simulink model "controllore2_nonlineare_con_gravita"  (R2022b)
settings: Solver=VariableStepAuto  StartTime=0.0  StopTime=10.0  RelTol=1e-3
settings Model: Creator=Antonio Montalto  LastModifiedBy=natal

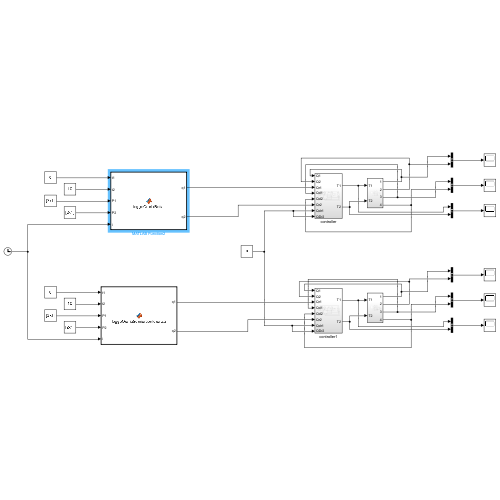
[thumbnail: Simulink's stored preview of the top-level diagram]
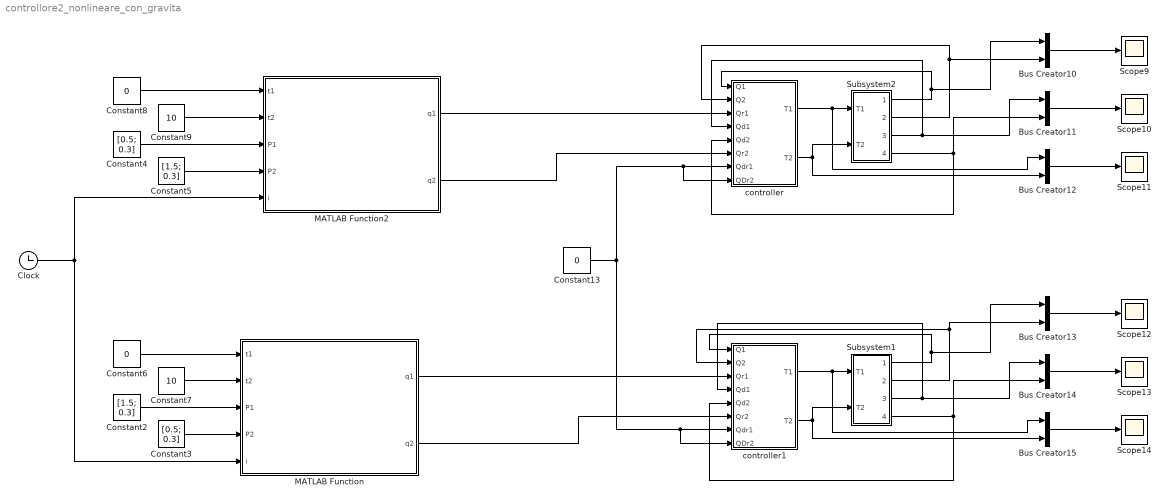
== system controllore2_nonlineare_con_gravita ==
  Bus Creator{10..15} (6 alike) : BusCreator  Inputs=2
  Clock : Clock
      settings: Decimation=1000
  Constant13 : Constant  Value=0
  Constant2 : Constant  Value=[1.5; 0.3]
  Constant3 : Constant  Value=[0.5; 0.3]
  Constant4 : Constant  Value=[0.5; 0.3]
  Constant5 : Constant  Value=[1.5; 0.3]
  Constant6 : Constant  Value=0
  Constant7 : Constant  Value=10
  Constant8 : Constant  Value=0
  Constant9 : Constant  Value=10
  MATLAB Function : MATLAB Function  TreatAsAtomicUnit=on
  MATLAB Function2 : MATLAB Function  TreatAsAtomicUnit=on
  Scope{9..14} (6 alike) : Scope
  Subsystem1 : Subsystem
  Subsystem2 : Subsystem
  controller : Subsystem
  controller1 : Subsystem
  wires:
  Bus Creator13/1 -> Scope12/1
  Subsystem2/1(Out1) -> controller/1(Q1), Bus Creator10/1
  controller1/2(T2) -> Subsystem1/2(T2), Bus Creator15/2
  Constant13/1 -> controller1/8(QDr2), controller1/7(Qdr1), controller/8(QDr2), controller/7(Qdr1)
  Subsystem1/3(Out3) -> controller1/4(Qd1), Bus Creator14/1
  Bus Creator14/1 -> Scope13/1
  Subsystem1/2(Out2) -> controller1/2(Q2), Bus Creator13/2
  Bus Creator15/1 -> Scope14/1
  Bus Creator11/1 -> Scope10/1
  controller1/1(T1) -> Subsystem1/1(T1), Bus Creator15/1
  Subsystem2/4(Out4) -> controller/5(Qd2), Bus Creator11/2
  Subsystem2/3(Out3) -> controller/4(Qd1), Bus Creator11/1
  Bus Creator10/1 -> Scope9/1
  controller/2(T2) -> Subsystem2/2(T2), Bus Creator12/2
  Subsystem1/4(Out4) -> controller1/5(Qd2), Bus Creator14/2
  Bus Creator12/1 -> Scope11/1
  Subsystem2/2(Out2) -> controller/2(Q2), Bus Creator10/2
  Subsystem1/1(Out1) -> controller1/1(Q1), Bus Creator13/1
  controller/1(T1) -> Subsystem2/1(T1), Bus Creator12/1
  Clock/1 -> MATLAB Function2/5(i), MATLAB Function/5(i)
  Constant5/1 -> MATLAB Function2/4(P2)
  Constant9/1 -> MATLAB Function2/2(t2)
  Constant2/1 -> MATLAB Function/3(P1)
  Constant6/1 -> MATLAB Function/1(t1)
  Constant4/1 -> MATLAB Function2/3(P1)
  Constant8/1 -> MATLAB Function2/1(t1)
  Constant7/1 -> MATLAB Function/2(t2)
  Constant3/1 -> MATLAB Function/4(P2)
  MATLAB Function2/1(q1) -> controller/3(Qr1)
  MATLAB Function2/2(q2) -> controller/6(Qr2)
  MATLAB Function/1(q1) -> controller1/3(Qr1)
  MATLAB Function/2(q2) -> controller1/6(Qr2)

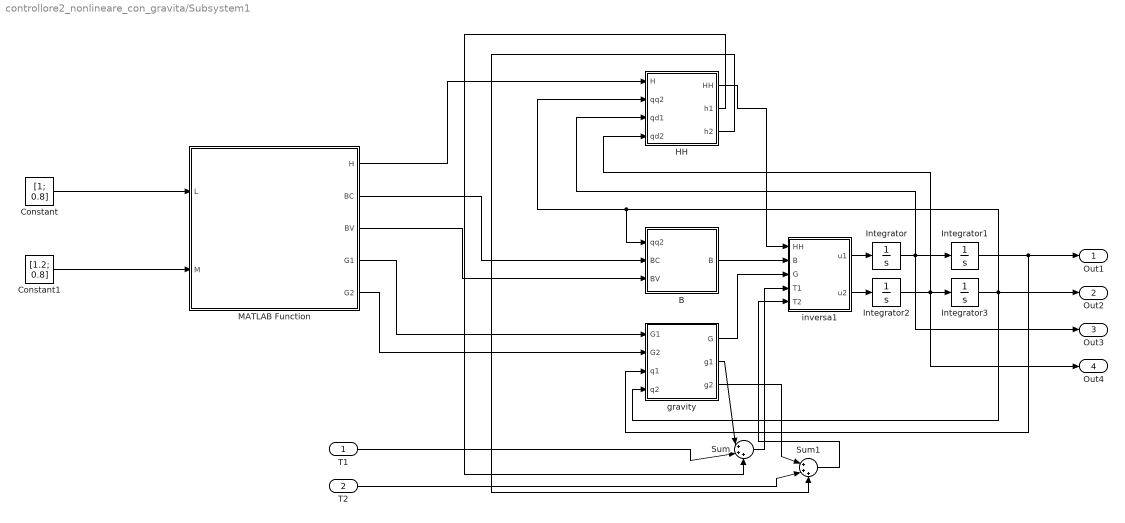
== system controllore2_nonlineare_con_gravita/Subsystem1 ==
  T1 : Inport
  T2 : Inport  Port=2
  B : MATLAB Function  TreatAsAtomicUnit=on
  Constant : Constant  Value=[1; 0.8]
  Constant1 : Constant  Value=[1.2; 0.8]
  HH : MATLAB Function  TreatAsAtomicUnit=on
  Integrator : Integrator
  Integrator1 : Integrator  InitialCondition=-1.7256
  Integrator2 : Integrator
  Integrator3 : Integrator  InitialCondition=2.5192
  MATLAB Function : MATLAB Function  TreatAsAtomicUnit=on
  Sum : Sum  Inputs=|+++
  Sum1 : Sum  Inputs=|+++
  gravity : MATLAB Function  TreatAsAtomicUnit=on
  inversa1 : MATLAB Function  TreatAsAtomicUnit=on
  Out1 : Outport
  Out2 : Outport  Port=2
  Out3 : Outport  Port=3
  Out4 : Outport  Port=4
  wires:
  Integrator2/1 -> Out4/1, Integrator3/1, HH/4(qd2)
  inversa1/1(u1) -> Integrator/1
  Integrator3/1 -> gravity/4(q2), Out2/1, HH/2(qq2), B/1(qq2)
  MATLAB Function/3(BV) -> B/3(BV)
  B/1(B) -> inversa1/2(B)
  Integrator/1 -> HH/3(qd1), Integrator1/1, Out3/1
  inversa1/2(u2) -> Integrator2/1
  HH/1(HH) -> inversa1/1(HH)
  MATLAB Function/1(H) -> HH/1(H)
  MATLAB Function/2(BC) -> B/2(BC)
  Integrator1/1 -> Out1/1, gravity/3(q1)
  gravity/1(G) -> inversa1/3(G)
  MATLAB Function/4(G1) -> gravity/1(G1)
  MATLAB Function/5(G2) -> gravity/2(G2)
  Constant/1 -> MATLAB Function/1(L)
  Constant1/1 -> MATLAB Function/2(M)
  T1/1 -> Sum/2
  T2/1 -> Sum1/2
  Sum/1 -> inversa1/4(T1)
  Sum1/1 -> inversa1/5(T2)
  gravity/2(g1) -> Sum/1
  gravity/3(g2) -> Sum1/1
  HH/2(h1) -> Sum/3
  HH/3(h2) -> Sum1/3

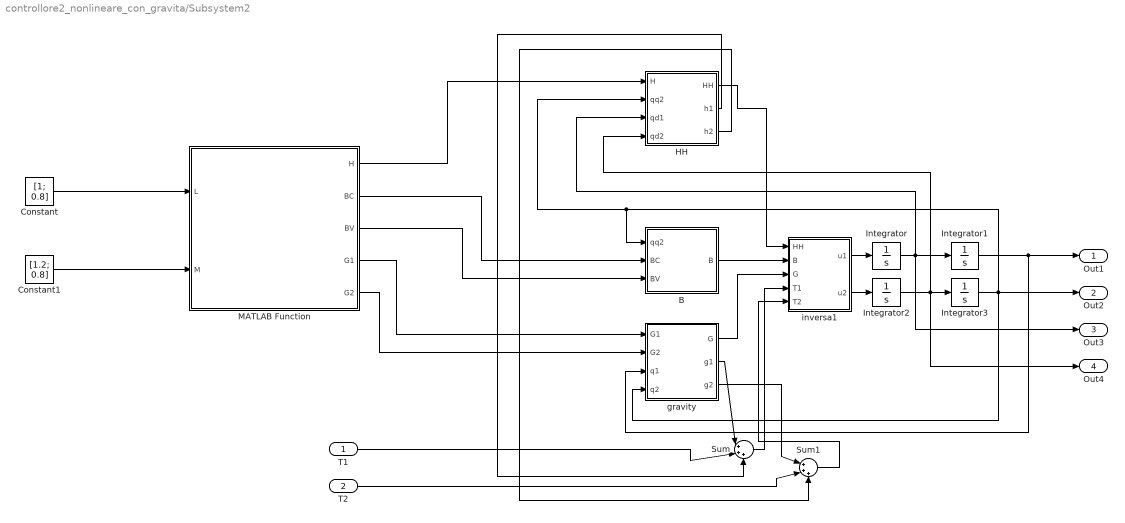
== system controllore2_nonlineare_con_gravita/Subsystem2 ==
  T1 : Inport
  T2 : Inport  Port=2
  B : MATLAB Function  TreatAsAtomicUnit=on
  Constant : Constant  Value=[1; 0.8]
  Constant1 : Constant  Value=[1.2; 0.8]
  HH : MATLAB Function  TreatAsAtomicUnit=on
  Integrator : Integrator
  Integrator1 : Integrator  InitialCondition=-1.7256
  Integrator2 : Integrator
  Integrator3 : Integrator  InitialCondition=2.5192
  MATLAB Function : MATLAB Function  TreatAsAtomicUnit=on
  Sum : Sum  Inputs=|+++
  Sum1 : Sum  Inputs=|+++
  gravity : MATLAB Function  TreatAsAtomicUnit=on
  inversa1 : MATLAB Function  TreatAsAtomicUnit=on
  Out1 : Outport
  Out2 : Outport  Port=2
  Out3 : Outport  Port=3
  Out4 : Outport  Port=4
  wires:
  Integrator2/1 -> Out4/1, Integrator3/1, HH/4(qd2)
  inversa1/1(u1) -> Integrator/1
  Integrator3/1 -> gravity/4(q2), Out2/1, HH/2(qq2), B/1(qq2)
  MATLAB Function/3(BV) -> B/3(BV)
  B/1(B) -> inversa1/2(B)
  Integrator/1 -> HH/3(qd1), Integrator1/1, Out3/1
  inversa1/2(u2) -> Integrator2/1
  HH/1(HH) -> inversa1/1(HH)
  MATLAB Function/1(H) -> HH/1(H)
  MATLAB Function/2(BC) -> B/2(BC)
  Integrator1/1 -> Out1/1, gravity/3(q1)
  gravity/1(G) -> inversa1/3(G)
  MATLAB Function/4(G1) -> gravity/1(G1)
  MATLAB Function/5(G2) -> gravity/2(G2)
  Constant/1 -> MATLAB Function/1(L)
  Constant1/1 -> MATLAB Function/2(M)
  T1/1 -> Sum/2
  T2/1 -> Sum1/2
  Sum/1 -> inversa1/4(T1)
  Sum1/1 -> inversa1/5(T2)
  gravity/2(g1) -> Sum/1
  gravity/3(g2) -> Sum1/1
  HH/2(h1) -> Sum/3
  HH/3(h2) -> Sum1/3

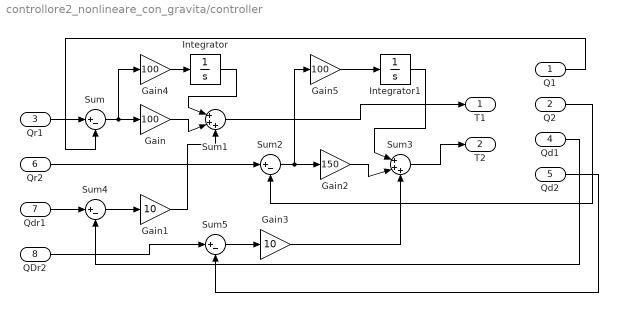
== system controllore2_nonlineare_con_gravita/controller ==
  Q1 : Inport
  Q2 : Inport  Port=2
  Qr1 : Inport  Port=3
  Qd1 : Inport  Port=4
  Qd2 : Inport  Port=5
  Qr2 : Inport  Port=6
  Qdr1 : Inport  Port=7
  QDr2 : Inport  Port=8
  Gain : Gain  Gain=100
  Gain1 : Gain  Gain=10
  Gain2 : Gain  Gain=150
  Gain3 : Gain  Gain=10
  Gain4 : Gain  Gain=100
  Gain5 : Gain  Gain=100
  Integrator : Integrator
  Integrator1 : Integrator
  Sum{,2,4..5} (4 alike) : Sum  Inputs=|+-
  Sum1 : Sum  Inputs=|+++
  Sum3 : Sum  Inputs=|+++
  T1 : Outport
  T2 : Outport  Port=2
  wires:
  Qd1/1 -> Sum4/2
  Sum/1 -> Gain4/1, Gain/1
  Gain/1 -> Sum1/2
  Gain2/1 -> Sum3/2
  Gain3/1 -> Sum3/3
  Sum2/1 -> Gain5/1, Gain2/1
  Q2/1 -> Sum2/2
  Qd2/1 -> Sum5/2
  Qr2/1 -> Sum2/1
  Sum3/1 -> T2/1
  Sum1/1 -> T1/1
  Qr1/1 -> Sum/1
  Q1/1 -> Sum/2
  Qdr1/1 -> Sum4/1
  Sum4/1 -> Gain1/1
  Gain1/1 -> Sum1/3
  QDr2/1 -> Sum5/1
  Sum5/1 -> Gain3/1
  Gain4/1 -> Integrator/1
  Integrator/1 -> Sum1/1
  Integrator1/1 -> Sum3/1
  Gain5/1 -> Integrator1/1

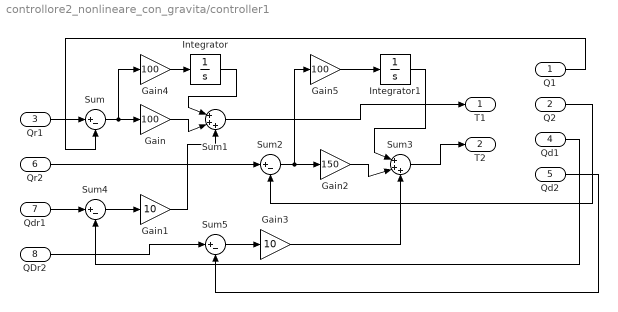
== system controllore2_nonlineare_con_gravita/controller1 ==
  Q1 : Inport
  Q2 : Inport  Port=2
  Qr1 : Inport  Port=3
  Qd1 : Inport  Port=4
  Qd2 : Inport  Port=5
  Qr2 : Inport  Port=6
  Qdr1 : Inport  Port=7
  QDr2 : Inport  Port=8
  Gain : Gain  Gain=100
  Gain1 : Gain  Gain=10
  Gain2 : Gain  Gain=150
  Gain3 : Gain  Gain=10
  Gain4 : Gain  Gain=100
  Gain5 : Gain  Gain=100
  Integrator : Integrator
  Integrator1 : Integrator
  Sum{,2,4..5} (4 alike) : Sum  Inputs=|+-
  Sum1 : Sum  Inputs=|+++
  Sum3 : Sum  Inputs=|+++
  T1 : Outport
  T2 : Outport  Port=2
  wires:
  Qd1/1 -> Sum4/2
  Sum/1 -> Gain4/1, Gain/1
  Gain/1 -> Sum1/2
  Gain2/1 -> Sum3/2
  Gain3/1 -> Sum3/3
  Sum2/1 -> Gain5/1, Gain2/1
  Q2/1 -> Sum2/2
  Qd2/1 -> Sum5/2
  Qr2/1 -> Sum2/1
  Sum3/1 -> T2/1
  Sum1/1 -> T1/1
  Qr1/1 -> Sum/1
  Q1/1 -> Sum/2
  Qdr1/1 -> Sum4/1
  Sum4/1 -> Gain1/1
  Gain1/1 -> Sum1/3
  QDr2/1 -> Sum5/1
  Sum5/1 -> Gain3/1
  Gain4/1 -> Integrator/1
  Integrator/1 -> Sum1/1
  Integrator1/1 -> Sum3/1
  Gain5/1 -> Integrator1/1

== matlab function controllore2_nonlineare_con_gravita/Subsystem2/HH ==
  data: H input; qq2 input; HH output; qd1 input; qd2 input; h1 output; h2 output
function [HH, h1, h2] = fcn(H,qq2,qd1,qd2)
uu1=H*sin(qq2);
HH =uu1*[(2*qd1*qd2+qd2^2); -qd1^2];
h1 = HH(1);
h2 = HH(2);

== matlab function controllore2_nonlineare_con_gravita/Subsystem2/MATLAB Function ==
  data: H output; L input; BC output; M input; BV output; G1 output; G2 output
function [H, BC, BV, G1, G2] = dati(L, M)
a1=L(1);
a2=L(2);
m1=M(1);
m2=M(2);
% gravità
g=9.8;


l1=a1/2;
l2=a2/2;
I1=m1*a1^2/12;
I2=m2*a2^2/12;
bc11=I1+I2+m1*l1^2+m2*(a1^2+l2^2);
bc12=I2+m2*l2^2;
bc21=bc12;
bc22=m2*l2^2+I2;
BC=[bc11 bc12; bc21 bc22];
bv11=2*a1*m2*l2;
bv12=a1*m1*l2;
bv21=bv12;
bv22=0;
BV=[bv11 bv12; bv21 bv22];
H=-m2*a1*l2;
G1=(m1*l1+m2*a1)*g;
G2=m2*l2*g;

== matlab function controllore2_nonlineare_con_gravita/Subsystem2/gravity ==
  data: G1 input; G output; G2 input; q1 input; q2 input; g1 output; g2 output
function [G, g1, g2]  = fcn(G1,G2,q1,q2)
c1=cos(q1);
c12=cos(q1+q2);

G = [G1*c1+G2*c12; G2*c12];
g1 = G(1);
g2 = G(2);

== matlab function controllore2_nonlineare_con_gravita/Subsystem2/inversa1 ==
  data: HH input; u1 output; B input; G input; T1 input; u2 output; T2 input
function [u1,u2] = fcn(HH,B,G,T1,T2)

y =inv(B)*([T1;T2]-HH-G);
u1=y(1);
u2=y(2);

== matlab function controllore2_nonlineare_con_gravita/Subsystem1/B ==
  data: qq2 input; B output; BC input; BV input
function B = fcn(qq2,BC,BV)
B=BC+cos(qq2)*BV;

== matlab function controllore2_nonlineare_con_gravita/Subsystem1/HH ==
  data: H input; qq2 input; HH output; qd1 input; qd2 input; h1 output; h2 output
function [HH, h1, h2] = fcn(H,qq2,qd1,qd2)
uu1=H*sin(qq2);
HH =uu1*[(2*qd1*qd2+qd2^2); -qd1^2];
h1 = HH(1);
h2 = HH(2);

== matlab function controllore2_nonlineare_con_gravita/Subsystem1/MATLAB Function ==
  data: H output; L input; BC output; M input; BV output; G1 output; G2 output
function [H, BC, BV, G1, G2] = dati(L, M)
a1=L(1);
a2=L(2);
m1=M(1);
m2=M(2);
% gravità
g=9.8;


l1=a1/2;
l2=a2/2;
I1=m1*a1^2/12;
I2=m2*a2^2/12;
bc11=I1+I2+m1*l1^2+m2*(a1^2+l2^2);
bc12=I2+m2*l2^2;
bc21=bc12;
bc22=m2*l2^2+I2;
BC=[bc11 bc12; bc21 bc22];
bv11=2*a1*m2*l2;
bv12=a1*m1*l2;
bv21=bv12;
bv22=0;
BV=[bv11 bv12; bv21 bv22];
H=-m2*a1*l2;
G1=(m1*l1+m2*a1)*g;
G2=m2*l2*g;

== matlab function controllore2_nonlineare_con_gravita/Subsystem1/gravity ==
  data: G1 input; G output; G2 input; q1 input; q2 input; g1 output; g2 output
function [G, g1, g2]  = fcn(G1,G2,q1,q2)
c1=cos(q1);
c12=cos(q1+q2);

G = [G1*c1+G2*c12; G2*c12];
g1 = G(1);
g2 = G(2);

== matlab function controllore2_nonlineare_con_gravita/Subsystem1/inversa1 ==
  data: HH input; u1 output; B input; G input; T1 input; u2 output; T2 input
function [u1,u2] = fcn(HH,B,G,T1,T2)

y =inv(B)*([T1;T2]-HH-G);
u1=y(1);
u2=y(2);

== matlab function controllore2_nonlineare_con_gravita/MATLAB Function ==
  data: t1 input; q1 output; t2 input; P1 input; P2 input; i input; q2 output
function [q1, q2] = leggeOrariaSemicirconferenza(t1, t2, P1, P2, i)
L = [1.0; 0.8];
Q1 = twolink_inverse(L, P1(1), P1(2));
Q2 = twolink_inverse(L, P2(1), P2(2));
lambda = calcolaLambda(calcolaSigma(t1, t2, i));
q1 = Q1(1) + lambda * (Q2(1) - Q1(1));
q2 = Q1(2) + lambda * (Q2(2) - Q1(2));
end

function Q = twolink_inverse(L, x, y)
L1 = L(1);
L2 = L(2);
Px = x;
Py = y;
P = [Px; Py];
c2 = (Px^2+Py^2-L1^2-L2^2)/(2*L1*L2);
s2 = sqrt(1-c2^2);
z = (1/(L1^2+L2^2+2*L1*L2*c2))*[L1+L2*c2 L2*s2; -L2*s2 L1+L2*c2]*P;
c1 = z(1, 1);
s1 = z(2, 1);
q1 = atan2(s1, c1);
q2 = atan2(s2, c2);
Q = [q1; q2];
end

function [sigma] = calcolaSigma(t1, t2, i)
sigma = (i-t1)/(t2-t1);
end

function [lambda] = calcolaLambda(sigma)
% lambda = -2*sigma^3 + 3*sigma^2;
% lambda = 6*sigma^5 - 15 *sigma^4 + 10*sigma^3;
lambda = -20*sigma^7 + 70*sigma^6 - 84*sigma^5 + 35*sigma^4;
end

== matlab function controllore2_nonlineare_con_gravita/MATLAB Function2 ==
  data: t1 input; q1 output; t2 input; P1 input; P2 input; i input; q2 output
function [q1, q2] = leggeOrariaRetta(t1, t2, P1, P2, i)
L = [1.0; 0.8];
lambda = calcolaLambda(calcolaSigma(t1, t2, i));
px = P1(1) + lambda*(P2(1) - P1(1));
py = P1(2) + lambda*(P2(2) - P1(2));
Q = twolink_inverse(L, px, py);
q1 = Q(1);
q2 = Q(2);
end

function Q = twolink_inverse(L, x, y)
L1 = L(1);
L2 = L(2);
Px = x;
Py = y;
P = [Px; Py];
c2 = (Px^2+Py^2-L1^2-L2^2)/(2*L1*L2);
s2 = sqrt(1-c2^2);
z = (1/(L1^2+L2^2+2*L1*L2*c2))*[L1+L2*c2 L2*s2; -L2*s2 L1+L2*c2]*P;
c1 = z(1, 1);
s1 = z(2, 1);
q1 = atan2(s1, c1);
q2 = atan2(s2, c2);
Q = [q1; q2];
end

function [sigma] = calcolaSigma(t1, t2, i)
sigma = (i-t1)/(t2-t1);
end

function [lambda] = calcolaLambda(sigma)
% lambda = -2*sigma^3 + 3*sigma^2;
% lambda = 6*sigma^5 - 15 *sigma^4 + 10*sigma^3;
lambda = -20*sigma^7 + 70*sigma^6 - 84*sigma^5 + 35*sigma^4;
end

== matlab function controllore2_nonlineare_con_gravita/Subsystem2/B ==
  data: qq2 input; B output; BC input; BV input
function B = fcn(qq2,BC,BV)
B=BC+cos(qq2)*BV;
